simulink model "a_downgrade"  (R2018a)
settings: Solver=VariableStepAuto  StartTime=0.0  StopTime=100  RelTol=1e-3
settings Model: Creator=aycfink  LastModifiedBy=aycfink
settings DebuggingCC: LibraryContextMissingDiagnostic=warning
settings SFSimCC: SimUseLocalCustomCode=on
settings RTWCC: RTWUseLocalCustomCode=on

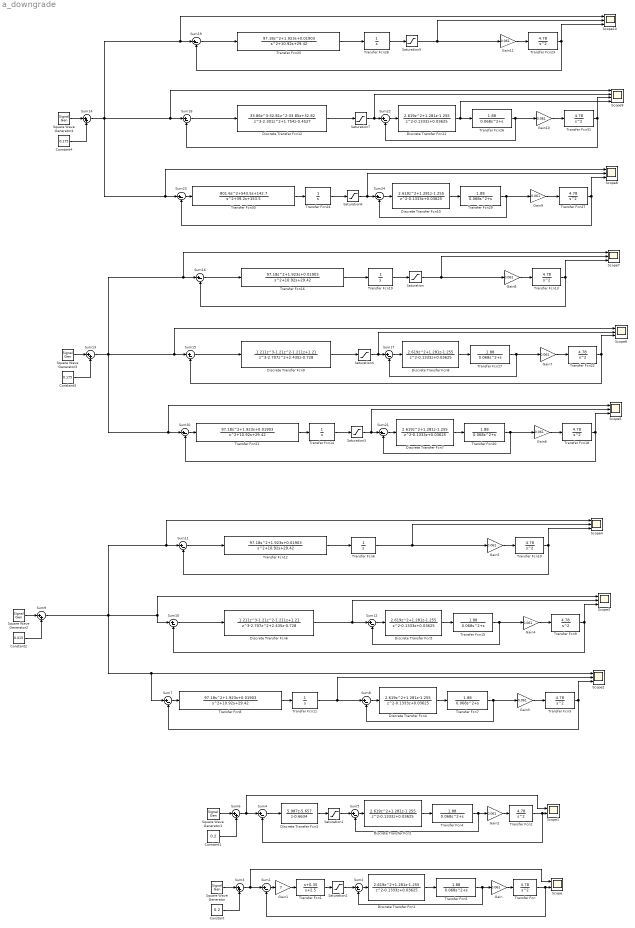
== system a_downgrade ==
  Constant : Constant  Value=0.2
  Constant1 : Constant  Value=0.2
  Constant2 : Constant  Value=0.015
  Constant3 : Constant  Value=0.175
  Constant4 : Constant  Value=0.175
  Discrete Transfer Fcn{1..2,4..5,7..8,10..11} (8 alike) : DiscreteTransferFcn  Numerator=[2.619 1.281 -1.255]  Denominator=[1 -0.1333 0.03625]  SampleTime=0.029012
  Discrete Transfer Fcn12 : DiscreteTransferFcn  Numerator=[33.86 -32.81 -33.85 32.82]  Denominator=[1 -2.301 1.754 -0.4527]  SampleTime=0.029012
  Discrete Transfer Fcn3 : DiscreteTransferFcn  Numerator=[5.987 -5.657]  Denominator=[1 -0.6634]  SampleTime=0.16186
  Discrete Transfer Fcn6 : DiscreteTransferFcn  Numerator=[1.211 -1.21 -1.211 1.21]  Denominator=[1 -2.707 2.435 -0.728]  SampleTime=0.029012
  Discrete Transfer Fcn9 : DiscreteTransferFcn  Numerator=[1.211 -1.21 -1.211 1.21]  Denominator=[1 -2.707 2.435 -0.728]  SampleTime=0.029012
  Gain{,2..11} (11 alike) : Gain  Gain=0.061
  Gain1 : Gain  Gain=7
  Saturation{,1..7} (8 alike) : Saturate  UpperLimit=0.7  LowerLimit=-0.7
  Scope : Scope  NumInputPorts=2
  Scope1 : Scope  NumInputPorts=2
  Scope{2..8,10} (8 alike) : Scope  NumInputPorts=3
  Scope9 : Scope  NumInputPorts=4
  Square Wave Generator : SignalGenerator  WaveForm=square  Amplitude=0.05  Frequency=0.2  Units=rad/sec
  Square Wave Generator1 : SignalGenerator  WaveForm=square  Amplitude=0.05  Frequency=0.2  Units=rad/sec
  Square Wave Generator2 : SignalGenerator  WaveForm=square  Amplitude=0.015  Frequency=0.2  Units=rad/sec
  Square Wave Generator3 : SignalGenerator  WaveForm=square  Amplitude=0.075  Frequency=0.2  Units=rad/sec
  Square Wave Generator4 : SignalGenerator  WaveForm=square  Amplitude=0.075  Frequency=0.2  Units=rad/sec
  Sum{1..2,4..5,7..8,10..12,15..24} (19 alike) : Sum  Inputs=|+-
  Sum{3,6,9,13..14} (5 alike) : Sum  Inputs=|++
  Transfer Fcn{,2..3,9..10,13,18,22..23,27,31} (11 alike) : TransferFcn  Numerator=[4.78]  Denominator=[1 0 0]
  Transfer Fcn1 : TransferFcn  Numerator=[1 0.35]  Denominator=[1 2.5]
  Transfer Fcn{6,11,14,19,24,28} (6 alike) : TransferFcn  Denominator=[1 0]
  Transfer Fcn{8,12,16,21,25} (5 alike) : TransferFcn  Numerator=[97.18 1.923 0.01903]  Denominator=[1 10.92 29.42]
  Transfer Fcn{4..5,7,15,17,20,26,29} (8 alike) : TransferFcn  Numerator=[1.88]  Denominator=[0.068 1 0]
  Transfer Fcn30 : TransferFcn  Numerator=[801.6 543.5 142.7]  Denominator=[1 39.2 153.5]
  wires:
  Saturation2/1 -> Sum2/1
  Transfer Fcn5/1 -> Sum2/2, Gain/1
  Discrete Transfer Fcn1/1 -> Transfer Fcn5/1
  Sum2/1 -> Discrete Transfer Fcn1/1
  Transfer Fcn1/1 -> Saturation2/1
  Gain/1 -> Transfer Fcn/1
  Transfer Fcn/1 -> Sum1/2, Scope/2
  Sum1/1 -> Gain1/1
  Gain1/1 -> Transfer Fcn1/1
  Square Wave Generator/1 -> Sum3/1
  Sum3/1 -> Scope/1, Sum1/1
  Constant/1 -> Sum3/2
  Sum6/1 -> Scope1/1, Sum4/1
  Square Wave Generator1/1 -> Sum6/1
  Sum5/1 -> Discrete Transfer Fcn2/1
  Transfer Fcn4/1 -> Sum5/2, Gain2/1
  Saturation1/1 -> Sum5/1
  Gain2/1 -> Transfer Fcn2/1
  Transfer Fcn2/1 -> Sum4/2, Scope1/2
  Discrete Transfer Fcn2/1 -> Transfer Fcn4/1
  Constant1/1 -> Sum6/2
  Sum4/1 -> Discrete Transfer Fcn3/1
  Discrete Transfer Fcn3/1 -> Saturation1/1
  Square Wave Generator2/1 -> Sum9/1
  Gain3/1 -> Transfer Fcn3/1
  Transfer Fcn3/1 -> Sum7/2, Scope2/3
  Constant2/1 -> Sum9/2
  Discrete Transfer Fcn4/1 -> Transfer Fcn7/1
  Transfer Fcn7/1 -> Sum8/2, Gain3/1
  Sum8/1 -> Discrete Transfer Fcn4/1
  Gain5/1 -> Transfer Fcn10/1
  Sum9/1 -> Sum10/1, Scope3/1, Scope4/1, Sum11/1, Sum7/1, Scope2/1
  Transfer Fcn10/1 -> Sum11/2, Scope4/3
  Discrete Transfer Fcn6/1 -> Scope3/2, Sum12/1
  Transfer Fcn9/1 -> Sum10/2, Scope3/3
  Gain4/1 -> Transfer Fcn9/1
  Transfer Fcn15/1 -> Sum12/2, Gain4/1
  Sum12/1 -> Discrete Transfer Fcn5/1
  Discrete Transfer Fcn5/1 -> Transfer Fcn15/1
  Sum10/1 -> Discrete Transfer Fcn6/1
  Sum11/1 -> Transfer Fcn12/1
  Sum7/1 -> Transfer Fcn8/1
  Transfer Fcn8/1 -> Transfer Fcn11/1
  Transfer Fcn11/1 -> Scope2/2, Sum8/1
  Transfer Fcn6/1 -> Scope4/2, Gain5/1
  Transfer Fcn12/1 -> Transfer Fcn6/1
  Transfer Fcn21/1 -> Transfer Fcn14/1
  Transfer Fcn16/1 -> Transfer Fcn19/1
  Sum16/1 -> Transfer Fcn16/1
  Sum20/1 -> Transfer Fcn21/1
  Transfer Fcn13/1 -> Sum16/2, Scope7/3
  Gain7/1 -> Transfer Fcn22/1
  Transfer Fcn22/1 -> Sum15/2, Scope6/3
  Discrete Transfer Fcn8/1 -> Transfer Fcn17/1
  Sum17/1 -> Discrete Transfer Fcn8/1
  Sum15/1 -> Discrete Transfer Fcn9/1
  Gain8/1 -> Transfer Fcn13/1
  Transfer Fcn17/1 -> Sum17/2, Gain7/1
  Transfer Fcn18/1 -> Sum20/2, Scope5/3
  Gain6/1 -> Transfer Fcn18/1
  Sum21/1 -> Discrete Transfer Fcn7/1
  Discrete Transfer Fcn7/1 -> Transfer Fcn20/1
  Transfer Fcn20/1 -> Sum21/2, Gain6/1
  Sum13/1 -> Scope5/1, Sum20/1, Scope7/1, Sum16/1, Scope6/1, Sum15/1
  Square Wave Generator3/1 -> Sum13/1
  Constant3/1 -> Sum13/2
  Discrete Transfer Fcn9/1 -> Saturation4/1
  Saturation4/1 -> Scope6/2, Sum17/1
  Transfer Fcn14/1 -> Saturation3/1
  Saturation3/1 -> Scope5/2, Sum21/1
  Transfer Fcn19/1 -> Saturation/1
  Saturation/1 -> Scope7/2, Gain8/1
  Transfer Fcn28/1 -> Saturation5/1
  Transfer Fcn24/1 -> Saturation6/1
  Saturation5/1 -> Scope10/2, Gain11/1
  Sum14/1 -> Scope8/1, Sum23/1, Scope10/1, Sum19/1, Scope9/1, Sum18/1
  Discrete Transfer Fcn10/1 -> Transfer Fcn29/1
  Gain9/1 -> Transfer Fcn27/1
  Transfer Fcn29/1 -> Sum24/2, Gain9/1
  Saturation6/1 -> Scope8/2, Sum24/1
  Gain11/1 -> Transfer Fcn23/1
  Sum24/1 -> Discrete Transfer Fcn10/1
  Sum18/1 -> Discrete Transfer Fcn12/1
  Transfer Fcn26/1 -> Gain10/1, Sum22/2
  Discrete Transfer Fcn11/1 -> Scope9/4, Transfer Fcn26/1
  Sum22/1 -> Discrete Transfer Fcn11/1
  Transfer Fcn31/1 -> Sum18/2, Scope9/3
  Saturation7/1 -> Scope9/2, Sum22/1
  Gain10/1 -> Transfer Fcn31/1
  Sum23/1 -> Transfer Fcn30/1
  Transfer Fcn30/1 -> Transfer Fcn24/1
  Square Wave Generator4/1 -> Sum14/1
  Transfer Fcn25/1 -> Transfer Fcn28/1
  Transfer Fcn27/1 -> Sum23/2, Scope8/3
  Sum19/1 -> Transfer Fcn25/1
  Discrete Transfer Fcn12/1 -> Saturation7/1
  Constant4/1 -> Sum14/2
  Transfer Fcn23/1 -> Sum19/2, Scope10/3
